simulink library "theta"  (Simulink 6.6)
settings Model: Creator=spaterna  LastModifiedBy=spaterna  ExtModeAutoUpdateStatusClock=off

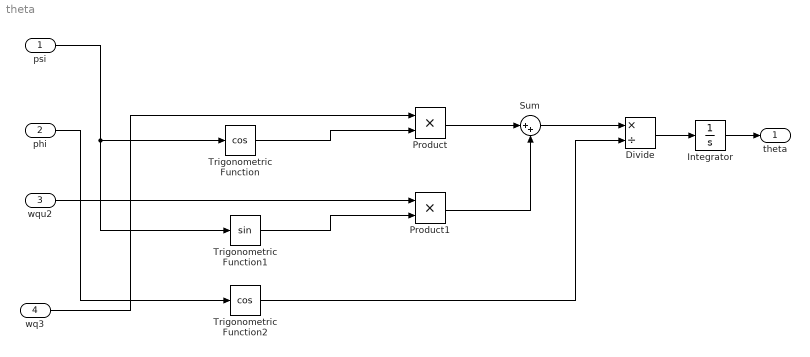
== system theta ==
  psi : Inport
  phi : Inport  Port=2
  wqu2 : Inport  Port=3
  wq3 : Inport  Port=4
  Divide : Product  Inputs=*/  OutScaling=2^-10
  Integrator : Integrator
  Product : Product  RndMeth=Zero
  Product1 : Product  RndMeth=Zero
  Sum : Sum  Inputs=|++
  Trigonometric Function : Trigonometry  Operator=cos
  Trigonometric Function1 : Trigonometry
  Trigonometric Function2 : Trigonometry  Operator=cos
  theta : Outport
  wires:
  wq3/1 -> Product/1
  wqu2/1 -> Product1/1
  Product/1 -> Sum/1
  Product1/1 -> Sum/2
  Sum/1 -> Divide/1
  Trigonometric Function2/1 -> Divide/2
  Divide/1 -> Integrator/1
  Trigonometric Function/1 -> Product/2
  Trigonometric Function1/1 -> Product1/2
  phi/1 -> Trigonometric Function2/1
  Integrator/1 -> theta/1
  psi/1 -> Trigonometric Function/1, Trigonometric Function1/1
